simulink model "model"  (R2024b)
settings: Solver=FixedStepAuto  StartTime=0  StopTime=12000  FixedStep=1  RelTol=1e-3
model workspace (MAT data in the model file):
  initial_altitude = 418
  initial_latitude = 48
  initial_longitude = 11
  updraft_locations = [48.9421342125 12.8571640345]
values from neighbouring files (symbols this model uses):
  sounding_buses = [sounding_buses, new_bus]    [create_bus.m]
  updrafts = cell(1, num_updrafts)    [test_thermal_model.m]
libraries: matrix_library x2, aerolibtransform2 x2, aerolibanim x1
settings Model: Creator=ge59guz  LastModifiedBy=Pedro
settings DebuggingCC: UnconnectedInputMsg=warning  UnconnectedOutputMsg=warning  UnconnectedLineMsg=warning
settings ModelReferenceCC: EnableRefExpFcnMdlSchedulingChecks=on
settings SFSimCC: LegacyBehaviorForPersistentVarInContinuousTime=on
settings RTWCC: GPUComputeCapability=3.5  DLArmComputeVersion=19.05

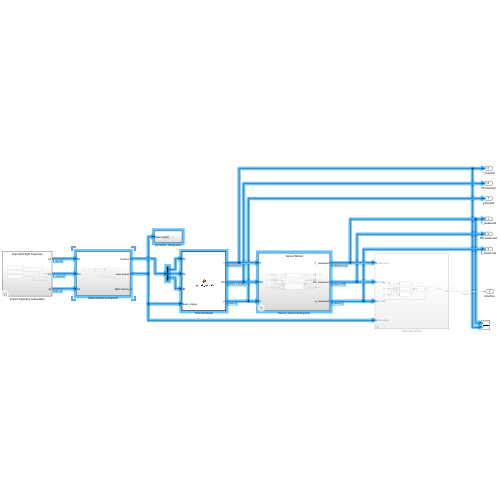
[thumbnail: Simulink's stored preview of the top-level diagram]
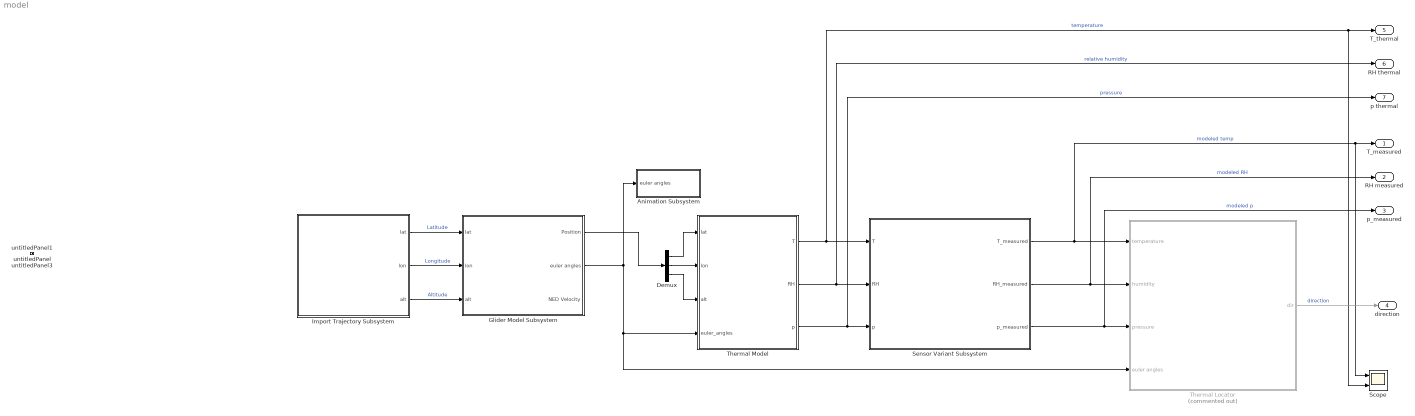
== system model ==
  Animation Subsystem : Subsystem
  Demux : Demux  Outputs=3
  Glider Model Subsystem : Subsystem
  Import Trajectory Subsystem : Subsystem  Variant=on
  Scope : Scope  NumInputPorts=2
  Sensor Variant Subsystem : Subsystem  Variant=on
  Thermal Locator : Subsystem  Commented=on
  Thermal Model : MATLAB Function  TreatAsAtomicUnit=on
  untitledPanel : Subsystem  Tag=HiddenForWebPanel  IsWebBlockPanel=on
  untitledPanel1 : Subsystem  Tag=HiddenForWebPanel  IsWebBlockPanel=on
  untitledPanel3 : Subsystem  Tag=HiddenForWebPanel  IsWebBlockPanel=on
  T_measured : Outport
  RH measured : Outport  Port=2
  p_measured : Outport  Port=3
  direction : Outport  Port=4
  T_thermal : Outport  Port=5
  RH thermal : Outport  Port=6
  p thermal : Outport  Port=7
  wires:
  Thermal Model/1(T) -> Sensor Variant Subsystem/1(T), Scope/2, T_thermal/1  "temperature"
  Thermal Model/3(p) -> p thermal/1, Sensor Variant Subsystem/3(p)  "pressure"
  Import Trajectory Subsystem/1(lat) -> Glider Model Subsystem/1(lat)  "Latitude"
  Import Trajectory Subsystem/2(lon) -> Glider Model Subsystem/2(lon)  "Longitude"
  Sensor Variant Subsystem/1(T_measured) -> Thermal Locator/1(temperature), Scope/1, T_measured/1  "modeled temp"
  Sensor Variant Subsystem/2(RH_measured) -> Thermal Locator/2(humidity), RH measured/1  "modeled RH"
  Sensor Variant Subsystem/3(p_measured) -> Thermal Locator/3(pressure), p_measured/1  "modeled p"
  Thermal Model/2(RH) -> Sensor Variant Subsystem/2(RH), RH thermal/1  "relative humidity"
  Import Trajectory Subsystem/3(alt) -> Glider Model Subsystem/3(alt)  "Altitude"
  Glider Model Subsystem/2(euler angles) -> Animation Subsystem/1(euler angles), Thermal Locator/4(euler angles), Thermal Model/4(euler_angles)
  Glider Model Subsystem/1(Position) -> Demux/1
  Demux/1 -> Thermal Model/1(lat)
  Demux/2 -> Thermal Model/2(lon)
  Demux/3 -> Thermal Model/3(alt)
  Thermal Locator/1(dir) -> direction/1  "direction"

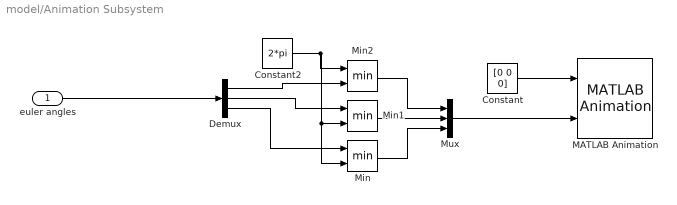
== system model/Animation Subsystem ==
  euler angles : Inport
  Constant : Constant  Value=[0 0 0]
  Constant2 : Constant  Value=2*pi
  Demux : Demux  Outputs=3
  MATLAB Animation : aerolibanim/MATLAB Animation  Tag=Matlab Animation 6 DOF  Vehicles=1  Geometries='pa24-250_orange.ac'  BoundingBoxCoordinates=[-50,50,-50,50,-50,50]  CameraOffset=[-150,-50,0]  CameraViewAngle=3  SampleTime=2  FigurePosition=[6.416667e+02,3.616667e+02,6.386667e+02,3.033333e+02]
  Min : MinMax  Inputs=2
  Min1 : MinMax  Inputs=2
  Min2 : MinMax  Inputs=2
  Mux : Mux  Inputs=3
  wires:
  Demux/3 -> Min/1
  Demux/2 -> Min1/1
  Demux/1 -> Min2/2
  Min2/1 -> Mux/1
  Min/1 -> Mux/3
  Min1/1 -> Mux/2
  euler angles/1 -> Demux/1
  Constant2/1 -> Min/2, Min1/2, Min2/1
  Constant/1 -> MATLAB Animation/1
  Mux/1 -> MATLAB Animation/2

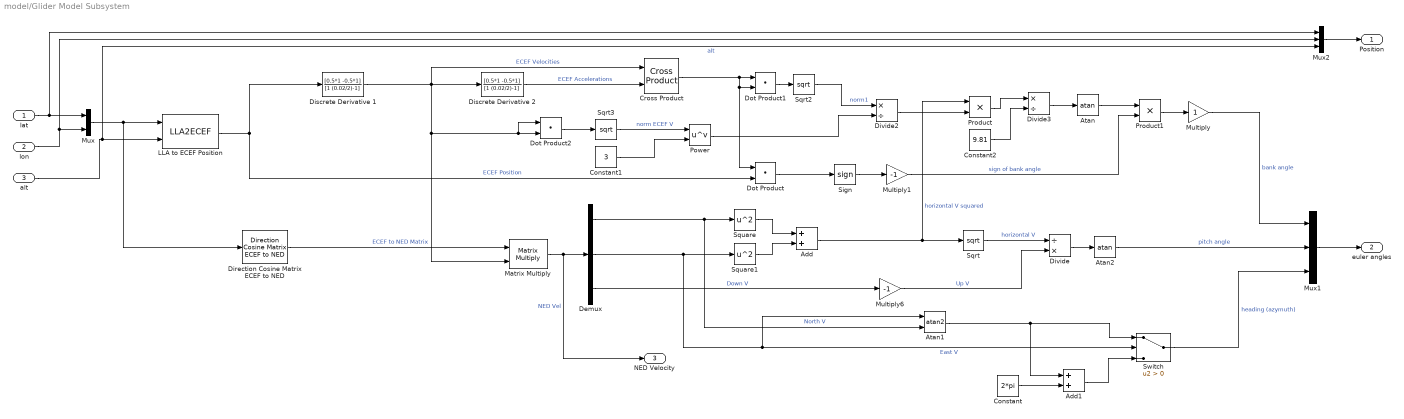
== system model/Glider Model Subsystem ==
  lat : Inport
  lon : Inport  Port=2
  alt : Inport  Port=3
  Add : Sum
  Add1 : Sum
  Atan : Trigonometry  Operator=atan
  Atan1 : Trigonometry  Operator=atan2
  Atan2 : Trigonometry  Operator=atan
  Constant : Constant  Value=2*pi
  Constant1 : Constant  Value=3
  Constant2 : Constant  Value=9.81
  Cross Product : matrix_library/Cross Product
  Demux : Demux  Outputs=3
  Direction Cosine Matrix ECEF to NED : aerolibtransform2/Direction Cosine Matrix ECEF to NED
  Discrete Derivative 1 : DiscreteTransferFcn  Numerator=[0.5*1 -0.5*1]  Denominator=[1 (0.02/2)-1]
  Discrete Derivative 2 : DiscreteTransferFcn  Numerator=[0.5*1 -0.5*1]  Denominator=[1 (0.02/2)-1]
  Divide : Product  Inputs=/*
  Divide2 : Product  Inputs=*/
  Divide3 : Product  Inputs=*/
  Dot Product : DotProduct  OutDataTypeStr=Inherit: Inherit via internal rule
  Dot Product1 : DotProduct  OutDataTypeStr=Inherit: Inherit via internal rule
  Dot Product2 : DotProduct  OutDataTypeStr=Inherit: Inherit via internal rule
  LLA to ECEF Position : LLA2ECEF
  Matrix Multiply : Product  Multiplication=Matrix(*)
  Multiply : Gain
  Multiply1 : Gain  Gain=-1
  Multiply6 : Gain  Gain=-1
  Mux : Mux  Inputs=2
  Mux1 : Mux  Inputs=3
  Mux2 : Mux  Inputs=3
  Power : Math  Operator=pow
  Product : Product
  Product1 : Product
  Sign : Signum
  Sqrt : Sqrt
  Sqrt2 : Sqrt
  Sqrt3 : Sqrt
  Square : Math  Operator=square
  Square1 : Math  Operator=square
  Switch : Switch  Criteria=u2 > Threshold  SaturateOnIntegerOverflow=off  InputSameDT=off
  Position : Outport
  euler angles : Outport  Port=2
  NED Velocity : Outport  Port=3
  wires:
  lon/1 -> Mux2/2, Mux/2
  lat/1 -> Mux2/1, Mux/1
  Mux/1 -> Direction Cosine Matrix ECEF to NED/1, LLA to ECEF Position/1
  alt/1 -> Mux2/3, LLA to ECEF Position/2  "alt"
  Direction Cosine Matrix ECEF to NED/1 -> Matrix Multiply/1  "ECEF to NED Matrix"
  LLA to ECEF Position/1 -> Dot Product/2, Discrete Derivative 1/1  "ECEF Position"
  Discrete Derivative 1/1 -> Matrix Multiply/2, Dot Product2/1, Dot Product2/2, Discrete Derivative 2/1, Cross Product/1  "ECEF Velocities"
  Matrix Multiply/1 -> NED Velocity/1, Demux/1  "NED Vel"
  Demux/2 -> Square1/1, Atan1/1, Switch/2  "East V"
  Demux/1 -> Atan1/2, Square/1  "North V"
  Square/1 -> Add/1
  Add/1 -> Sqrt/1, Product/1  "horizontal V squared"
  Cross Product/1 -> Dot Product/1, Dot Product1/2, Dot Product1/1
  Dot Product2/1 -> Sqrt3/1
  Sqrt3/1 -> Power/1  "norm ECEF V"
  Constant1/1 -> Power/2
  Sqrt2/1 -> Divide2/1  "norm1"
  Power/1 -> Divide2/2
  Divide2/1 -> Product/2
  Product/1 -> Divide3/1
  Constant2/1 -> Divide3/2
  Divide3/1 -> Atan/1
  Atan/1 -> Product1/1
  Multiply/1 -> Mux1/1  "bank angle"
  Dot Product/1 -> Sign/1
  Sign/1 -> Multiply1/1
  Product1/1 -> Multiply/1
  Dot Product1/1 -> Sqrt2/1
  Multiply1/1 -> Product1/2  "sign of bank angle"
  Square1/1 -> Add/2
  Constant/1 -> Add1/2
  Atan1/1 -> Add1/1, Switch/1
  Add1/1 -> Switch/3
  Switch/1 -> Mux1/3  "heading (azymuth)"
  Sqrt/1 -> Divide/1  "horizontal V"
  Divide/1 -> Atan2/1
  Demux/3 -> Multiply6/1  "Down V"
  Atan2/1 -> Mux1/2  "pitch angle"
  Multiply6/1 -> Divide/2  "Up V"
  Mux1/1 -> euler angles/1
  Discrete Derivative 2/1 -> Cross Product/2  "ECEF Accelerations"
  Mux2/1 -> Position/1

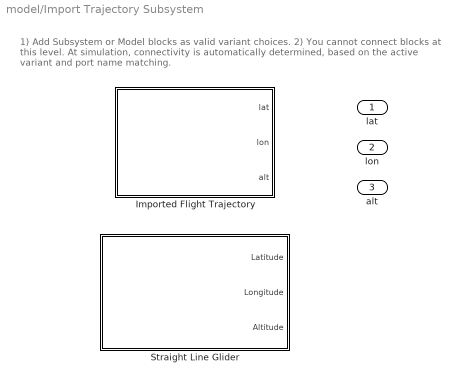
== system model/Import Trajectory Subsystem ==
  note: 1) Add Subsystem or Model blocks as valid variant choices.
      | 2) You cannot connect blocks at this level. At simulation, connectivity is automatically
      | determined, based on the active variant and port name matching.
  Imported Flight Trajectory : Subsystem  VariantControl=true
  Straight Line Glider : Subsystem  VariantControl=false
  lat : Outport
  lon : Outport  Port=2
  alt : Outport  Port=3

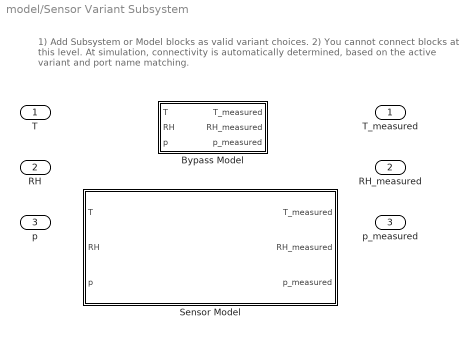
== system model/Sensor Variant Subsystem ==
  note: 1) Add Subsystem or Model blocks as valid variant choices.
      | 2) You cannot connect blocks at this level. At simulation, connectivity is automatically
      | determined, based on the active variant and port name matching.
  T : Inport
  RH : Inport  Port=2
  p : Inport  Port=3
  Bypass Model : Subsystem  VariantControl=false
  Sensor Model : Subsystem  VariantControl=true
  T_measured : Outport
  RH_measured : Outport  Port=2
  p_measured : Outport  Port=3

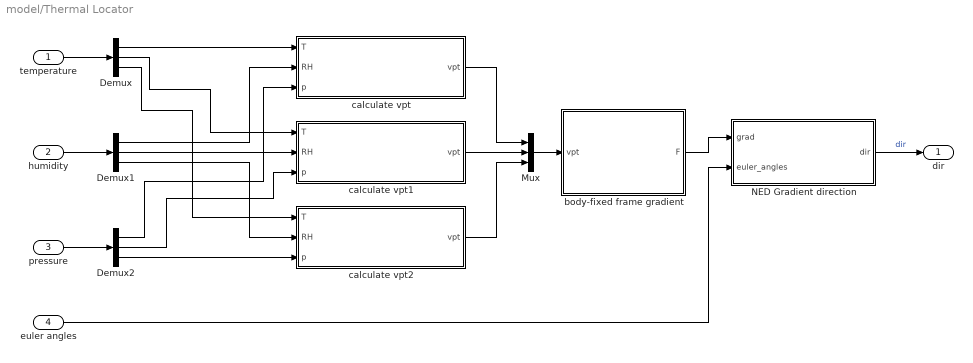
== system model/Thermal Locator ==
  temperature : Inport
  humidity : Inport  Port=2
  pressure : Inport  Port=3
  euler angles : Inport  Port=4
  Demux : Demux  Outputs=3
  Demux1 : Demux  Outputs=3
  Demux2 : Demux  Outputs=3
  Mux : Mux  Inputs=3
  NED Gradient direction : MATLAB Function  TreatAsAtomicUnit=on
  body-fixed frame gradient : MATLAB Function  TreatAsAtomicUnit=on
  calculate vpt : MATLAB Function  TreatAsAtomicUnit=on
  calculate vpt1 : MATLAB Function  TreatAsAtomicUnit=on
  calculate vpt2 : MATLAB Function  TreatAsAtomicUnit=on
  dir : Outport
  wires:
  temperature/1 -> Demux/1
  Demux/1 -> calculate vpt/1(T)
  Demux/2 -> calculate vpt1/1(T)
  Demux/3 -> calculate vpt2/1(T)
  humidity/1 -> Demux1/1
  Demux1/1 -> calculate vpt/2(RH)
  Demux1/2 -> calculate vpt1/2(RH)
  Demux1/3 -> calculate vpt2/2(RH)
  pressure/1 -> Demux2/1
  Demux2/1 -> calculate vpt/3(p)
  Demux2/2 -> calculate vpt1/3(p)
  Demux2/3 -> calculate vpt2/3(p)
  calculate vpt/1(vpt) -> Mux/1
  calculate vpt1/1(vpt) -> Mux/2
  calculate vpt2/1(vpt) -> Mux/3
  Mux/1 -> body-fixed frame gradient/1(vpt)
  body-fixed frame gradient/1(F) -> NED Gradient direction/1(grad)
  euler angles/1 -> NED Gradient direction/2(euler_angles)
  NED Gradient direction/1(dir) -> dir/1  "dir"

== system model/untitledPanel ==
  panelInfo : PanelWebBlock  Tag=HiddenForWebPanel  PanelInfo="{\"compacted\":true,\"height\":246,\"isActiveTab\":false,\"labels\":{\"label1365784696\":{\"deleted\":false,\"left\":18,\"settings\":{\"backgroundColor\":\"rgba(0, 0, 0, 0)\",\"bold\":false,\"font\":\"Arial\",\"fontColor\":\"black\",\"fontSize\":0.91,\"italicized\":false,\"underlined\":false},\"text\":\"Lifting condensation level:\",\"top\":138},\"label2522607047\":{\"deleted\":false,\"left\":20,\"settings\":{\"backgroundColor\":\"rgba(0, 0, 0, 0)\",\"bold\":false,\"font\":\"Arial\",\"fontColor\":\"black\",\"fontSize\":0.91,\"italicized\":false,\"underlined\":false},\"text\":\"Sounding location:\",\"top\":61},\"label6819632646\":{\"deleted\":false,\"left\":18,\"settings\":{\"backgroundColor\":\"rgba(0, 0, 0, 0)\",\"bold\":false,\"font\":\"Arial\",\"fontColor\":\"black\",\"fontSize\":0.91,\"italicized\":false,\"underlined\":false},\"text\":\"Mixed layer height:\",\"top\":100},\"label7929561413\":{\"deleted\":false,\"left\":18,\"settings\":{\"backgroundColor\":\"rgba(0, 0, 0, 0)\",\"bold\":false,\"font\":\"Arial\",\"fontColor\":\"black\",\"fontSize\":0.91,\"italicized\":false,\"underlined\":false},\"text\":\"Sounding date:\",\"top\":22}},\"left\":1938,\"name\":\"Sounding\",\"panelId\":\"panelId-b7bbacb4-b1f5-40a6-a59f-f1281bc15f19\",\"tabIndex\":2,\"tabbedSetId\":\"tabbedSet2696921389\",\"top\":7,\"type\":\"panel\",\"version\":\"2019b\",\"visible\":false,\"width\":464,\"zIndex\":1500006}"  PanelSnapshot=<binary blob, 23204 chars, not shown>

== system model/untitledPanel1 ==
  Climb : EditField  Tag=HiddenForWebPanel  PanelInfo="{\"height\":33,\"left\":126,\"panelId\":\"panelId-a8974220-6362-43f7-be10-4c2880e9e60b\",\"top\":107,\"type\":\"panelChild\",\"version\":\"2019b\",\"width\":46,\"zIndex\":1500006}"  LabelPosition=Hide  ShowInitialText=on  Alignment=Center
  Heading : EditField  Tag=HiddenForWebPanel  PanelInfo="{\"height\":31,\"left\":125,\"panelId\":\"panelId-a8974220-6362-43f7-be10-4c2880e9e60b\",\"top\":69,\"type\":\"panelChild\",\"version\":\"2019b\",\"width\":46,\"zIndex\":1500004}"  LabelPosition=Hide  ShowInitialText=on  Alignment=Center
  panelInfo : PanelWebBlock  Tag=HiddenForWebPanel  PanelInfo="{\"compacted\":true,\"height\":223,\"isActiveTab\":true,\"labels\":{\"label0009524542\":{\"deleted\":false,\"left\":132,\"settings\":{\"backgroundColor\":\"rgba(0, 0, 0, 0)\",\"bold\":false,\"font\":\"Arial\",\"fontColor\":\"black\",\"fontSize\":0.82,\"italicized\":false,\"underlined\":false},\"text\":\"alt\",\"top\":167},\"label0163547761\":{\"deleted\":false,\"left\":23,\"settings\":{\"backgroundColor\":\"rgba(0, 0, 0, 0)\",\"bold\":false,\"font\":\"Arial\",\"fontColor\":\"black\",\"fontSize\":0.82,\"italicized\":false,\"underlined\":false},\"text\":\"lat\",\"top\":167},\"label2478146783\":{\"deleted\":false,\"left\":11,\"settings\":{\"backgroundColor\":\"rgba(0, 0, 0, 0)\",\"bold\":false,\"font\":\"Arial\",\"fontColor\":\"black\",\"fontSize\":0.82,\"italicized\":false,\"underlined\":false},\"text\":\"climb angle (deg)\",\"top\":116},\"label4468598914\":{\"deleted\":false,\"left\":10,\"settings\":{\"backgroundColor\":\"rgba(0, 0, 0, 0)\",\"bold\":false,\"font\":\"Arial\",\"fontColor\":\"black\",\"fontSize\":0.82,\"italicized\":false,\"underlined\":false},\"text\":\"heading (deg)\",\"top\":77},\"label4953567006\":{\"deleted\":false,\"left\":9,\"settings\":{\"backgroundColor\":\"rgba(0, 0, 0, 0)\",\"bold\":false,\"font\":\"Arial\",\"fontColor\":\"black\",\"fontSize\":0.82,\"italicized\":false,\"underlined\":false},\"text\":\"initial velocity (m\\/s)\",\"top\":39},\"label6880872590\":{\"deleted\":false,\"left\":74,\"settings\":{\"backgroundColor\":\"rgba(0, 0, 0, 0)\",\"bold\":false,\"font\":\"Arial\",\"fontColor\":\"black\",\"fontSize\":0.82,\"italicized\":false,\"underlined\":false},\"text\":\"lon\",\"top\":167},\"label9788082855\":{\"deleted\":false,\"left\":12,\"settings\":{\"backgroundColor\":\"rgba(0, 0, 0, 0)\",\"bold\":true,\"font\":\"Arial\",\"fontColor\":\"black\",\"fontSize\":0.82,\"italicized\":false,\"underlined\":false},\"text\":\"Inputs\",\"top\":9},\"label9797548924\":{\"deleted\":false,\"left\":13,\"settings\":{\"backgroundColor\":\"rgba(0, 0, 0, 0)\",\"bold\":false,\"font\":\"Arial\",\"fontColor\":\"black\",\"fontSize\":0.82,\"italicized\":false,\"underlined\":false},\"text\":\"initial position (deg, m)\",\"top\":147}},\"left\":1938,\"name\":\"Glider\",\"panelId\":\"panelId-a8974220-6362-43f7-be10-4c2880e9e60b\",\"tabIndex\":0,\"tabbedSetId\":\"tabbedSet2696921389\",\"top\":7,\"type\":\"panel\",\"version\":\"2019b\",\"visible\":true,\"width\":484,\"zIndex\":1500004}"  PanelSnapshot=<binary blob, 27484 chars, not shown>
  velocity : EditField  Tag=HiddenForWebPanel  PanelInfo="{\"height\":33,\"left\":124,\"panelId\":\"panelId-a8974220-6362-43f7-be10-4c2880e9e60b\",\"top\":31,\"type\":\"panelChild\",\"version\":\"2019b\",\"width\":47,\"zIndex\":1500002}"  LabelPosition=Hide  ShowInitialText=on  Alignment=Center

== system model/untitledPanel3 ==
  Callback Button : CustomCallbackButton  Tag=HiddenForWebPanel  PanelInfo="{\"height\":50,\"left\":66,\"panelId\":\"panelId-5dd198ca-f2e6-4c37-9029-21f4a79994a1\",\"top\":24,\"type\":\"panelChild\",\"version\":\"2019b\",\"width\":142,\"zIndex\":1500002}"  Configuration="{\"components\":[{\"name\":\"BackgroundImageComponent\",\"settings\":{\"image\":{\"size\":[0,0],\"src\":\"default\",\"srcOrientation\":\"Right\"},\"position\":[0,0,1,1]}},{\"name\":\"ButtonStateComponent\",\"settings\":{\"buttonType\":\"momentary\",\"clickFcn\":\"[filename,filepath] = uigetfile({'*.igc';'*.mat'});\\n\\nif filename == 0\\n    return\\nelseif contains(filename, '.igc')\\n    % Parse igc file\\n    [flight, name] = parse_igc_file([filepath filename]);\\n    % Save flight to a .mat file\\n    save(strcat('Flights\\/',name, '.mat'), 'flight');\\nelseif contains(filename, '.mat')\\n    % Open saved flight\\n    load([filepath filename]);\\nelse\\n    return\\nend\\n\",\"latched\":false,\"offValue\":null,\"onValue\":1,\"position\":[0,0,1,1],\"pressDelay\":\"500\",\"pressFcn\":\"\",\"repeatInterval\":\"0\",\"states\":[{\"horizontalAlignment\":\"center\",\"image\":{\"position\":[0,0,1,1],\"size\":[1,1],\"src\":\"default\",\"srcOrientation\":\"Right\"},\"label\":{\"color\":[0.01176470588,0.01176470588,0.01176470588,1],\"icon\":{\"size\":[0,0],\"src\":\"default\",\"srcOrientation\":\"Right\"},\"iconPlacement\":\"left\",\"opacity\":1,\"show\":true,\"text\":{\"content\":\"Load flight\",\"font\":\"Helvetica\"}},\"labelOffset\":[0,0],\"verticalAlignment\":\"middle\"},{\"horizontalAlignment\":\"center\",\"image\":{\"position\":[0,0,1,1],\"size\":[1,1],\"src\":\"default\",\"srcOrientation\":\"Right\"},\"label\":{\"color\":[0.01176470588,0.01176470588,0.01176470588,1],\"icon\":{\"size\":[0,0],\"src\":\"default\",\"srcOrientation\":\"Right\"},\"iconPlacement\":\"left\",\"opacity\":1,\"show\":true,\"text\":{\"content\":\"Load flight\",\"font\":\"Helvetica\"}},\"labelOffset\":[0,0],\"verticalAlignment\":\"middle\"},{\"horizontalAlignment\":\"center\",\"image\":{\"position\":[0,0,1,1],\"size\":[1,1],\"src\":\"default\",\"srcOrientation\":\"Right\"},\"label\":{\"color\":[0.01176470588,0.01176470588,0.01176470588,1],\"icon\":{\"size\":[0,0],\"src\":\"default\",\"srcOrientation\":\"Right\"},\"iconPlacement\":\"left\",\"opacity\":1,\"show\":true,\"text\":{\"content\":\"Load flight\",\"font\":\"Helvetica\"}},\"labelOffset\":[0,0],\"verticalAlignment\":\"middle\"},{\"horizontalAlignment\":\"center\",\"image\":{\"position\":[0,0,1,1],\"size\":[1,1],\"src\":\"default\",\"srcOrientation\":\"Right\"},\"label\":{\"color\":[0.01176470588,0.01176470588,0.01176470588,1],\"icon\":{\"size\":[0,0],\"src\":\"default\",\"srcOrientation\":\"Right\"},\"iconPlacement\":\"left\",\"opacity\":1,\"show\":true,\"text\":{\"content\":\"Load flight\",\"font\":\"Helvetica\"}},\"labelOffset\":[0,0],\"verticalAlignment\":\"middle\"}]}},{\"name\":\"ForegroundImageComponent\",\"settings\":{\"image\":{\"size\":[0,0],\"src\":\"default\",\"srcOrientation\":\"Right\"},\"isForeground\":1,\"position\":[0,0,1,1]}}],\"settings\":{\"BindingType\":\"standalone\",\"backgroundColor\":[244,244,244,1],\"backgroundOffset\":0.2,\"backgroundOpacity\":1,\"fixedAspectRatio\":\"off\",\"foregroundColor\":[0.01176470588,0.01176470588,0.01176470588,1],\"migratedFromLegacy\":true,\"useBackgroundColor\":true,\"variant\":\"callback\",\"version\":\"R2024b\"},\"type\":\"Button\"}"  CustomBackgroundColor="{\"color\":[0.9568627451,0.9568627451,0.9568627451],\"show\":true}"
  Callback Button1 : CustomCallbackButton  Tag=HiddenForWebPanel  PanelInfo="{\"height\":47,\"left\":62,\"panelId\":\"panelId-5dd198ca-f2e6-4c37-9029-21f4a79994a1\",\"top\":89,\"type\":\"panelChild\",\"version\":\"2019b\",\"width\":149,\"zIndex\":1499998}"  Configuration="{\"components\":[{\"name\":\"BackgroundImageComponent\",\"settings\":{\"image\":{\"size\":[0,0],\"src\":\"default\",\"srcOrientation\":\"Right\"},\"position\":[0,0,1,1]}},{\"name\":\"ButtonStateComponent\",\"settings\":{\"buttonType\":\"momentary\",\"clickFcn\":\"display_chart(flight.trajectory,stations);\",\"onValue\":1,\"position\":[0,0,1,1],\"pressDelay\":\"500\",\"pressFcn\":\"\",\"repeatInterval\":\"0\",\"states\":[{\"horizontalAlignment\":\"center\",\"image\":{\"position\":[0,0,1,1],\"size\":[1,1],\"src\":\"default\",\"srcOrientation\":\"Right\"},\"label\":{\"color\":[0.01176470588,0.01176470588,0.01176470588,1],\"icon\":{\"size\":[0,0],\"src\":\"default\",\"srcOrientation\":\"Right\"},\"iconPlacement\":\"left\",\"opacity\":1,\"show\":true,\"text\":{\"content\":\"Place updrafts\",\"font\":\"Helvetica\"}},\"labelOffset\":[0,0],\"verticalAlignment\":\"middle\"},{\"horizontalAlignment\":\"center\",\"image\":{\"position\":[0,0,1,1],\"size\":[1,1],\"src\":\"default\",\"srcOrientation\":\"Right\"},\"label\":{\"color\":[0.01176470588,0.01176470588,0.01176470588,1],\"icon\":{\"size\":[0,0],\"src\":\"default\",\"srcOrientation\":\"Right\"},\"iconPlacement\":\"left\",\"opacity\":1,\"show\":true,\"text\":{\"content\":\"Place updrafts\",\"font\":\"Helvetica\"}},\"labelOffset\":[0,0],\"verticalAlignment\":\"middle\"},{\"horizontalAlignment\":\"center\",\"image\":{\"position\":[0,0,1,1],\"size\":[1,1],\"src\":\"default\",\"srcOrientation\":\"Right\"},\"label\":{\"color\":[0.01176470588,0.01176470588,0.01176470588,1],\"icon\":{\"size\":[0,0],\"src\":\"default\",\"srcOrientation\":\"Right\"},\"iconPlacement\":\"left\",\"opacity\":1,\"show\":true,\"text\":{\"content\":\"Place updrafts\",\"font\":\"Helvetica\"}},\"labelOffset\":[0,0],\"verticalAlignment\":\"middle\"},{\"horizontalAlignment\":\"center\",\"image\":{\"position\":[0,0,1,1],\"size\":[1,1],\"src\":\"default\",\"srcOrientation\":\"Right\"},\"label\":{\"color\":[0.01176470588,0.01176470588,0.01176470588,1],\"icon\":{\"size\":[0,0],\"src\":\"default\",\"srcOrientation\":\"Right\"},\"iconPlacement\":\"left\",\"opacity\":1,\"show\":true,\"text\":{\"content\":\"Place updrafts\",\"font\":\"Helvetica\"}},\"labelOffset\":[0,0],\"verticalAlignment\":\"middle\"}]}},{\"name\":\"ForegroundImageComponent\",\"settings\":{\"image\":{\"size\":[0,0],\"src\":\"default\",\"srcOrientation\":\"Right\"},\"isForeground\":1,\"position\":[0,0,1,1]}}],\"settings\":{\"BindingType\":\"standalone\",\"backgroundColor\":[244,244,244,1],\"backgroundOffset\":0.2,\"backgroundOpacity\":1,\"fixedAspectRatio\":\"off\",\"foregroundColor\":[0.01176470588,0.01176470588,0.01176470588,1],\"migratedFromLegacy\":true,\"useBackgroundColor\":true,\"variant\":\"callback\",\"version\":\"R2024b\"},\"type\":\"Button\"}"  CustomBackgroundColor="{\"color\":[0.9568627451,0.9568627451,0.9568627451],\"show\":true}"
  panelInfo : PanelWebBlock  Tag=HiddenForWebPanel  PanelInfo="{\"compacted\":true,\"height\":231,\"isActiveTab\":false,\"left\":1938,\"name\":\"Flight\",\"panelId\":\"panelId-5dd198ca-f2e6-4c37-9029-21f4a79994a1\",\"tabIndex\":1,\"tabbedSetId\":\"tabbedSet2696921389\",\"top\":7,\"type\":\"panel\",\"version\":\"2019b\",\"visible\":false,\"width\":437,\"zIndex\":1500010}"  PanelSnapshot=<binary blob, 11188 chars, not shown>

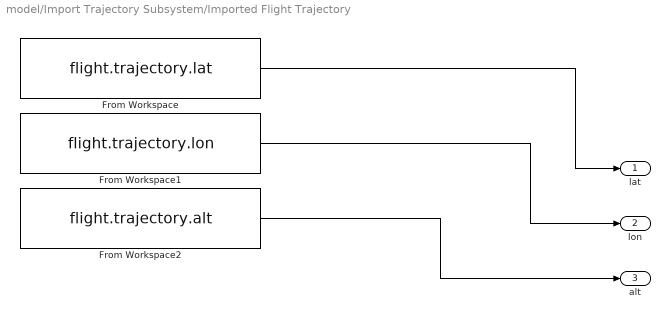
== system model/Import Trajectory Subsystem/Imported Flight Trajectory ==
  From Workspace : FromWorkspace  VariableName=flight.trajectory.lat  ZeroCross=off  OutputAfterFinalValue=Holding final value
  From Workspace1 : FromWorkspace  VariableName=flight.trajectory.lon  ZeroCross=off  OutputAfterFinalValue=Holding final value
  From Workspace2 : FromWorkspace  VariableName=flight.trajectory.alt  ZeroCross=off  OutputAfterFinalValue=Holding final value
  lat : Outport
  lon : Outport  Port=2
  alt : Outport  Port=3
  wires:
  From Workspace1/1 -> lon/1
  From Workspace/1 -> lat/1
  From Workspace2/1 -> alt/1

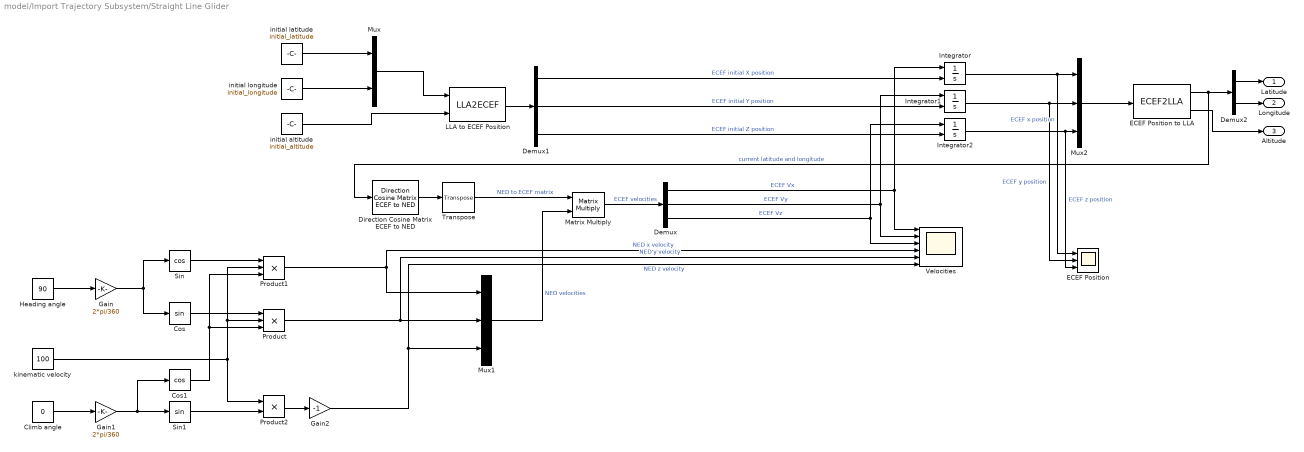
== system model/Import Trajectory Subsystem/Straight Line Glider ==
  Climb angle : Constant  Value=0
  Cos : Trigonometry  OutputSignalType=real
  Cos1 : Trigonometry  Operator=cos
  Demux : Demux  Outputs=3
  Demux1 : Demux  Outputs=3
  Demux2 : Demux  Outputs=2
  Direction Cosine Matrix ECEF to NED : aerolibtransform2/Direction Cosine Matrix ECEF to NED
  ECEF Position : Scope  NumInputPorts=3
  ECEF Position to LLA : ECEF2LLA
  Gain : Gain  Gain=2*pi/360
  Gain1 : Gain  Gain=2*pi/360
  Gain2 : Gain  Gain=-1
  Heading angle : Constant  Value=90
  Integrator : Integrator  InitialConditionSource=external
  Integrator1 : Integrator  InitialConditionSource=external
  Integrator2 : Integrator  InitialConditionSource=external
  LLA to ECEF Position : LLA2ECEF
  Matrix Multiply : Product  Multiplication=Matrix(*)
  Mux : Mux  Inputs=2
  Mux1 : Mux  Inputs=3
  Mux2 : Mux  Inputs=3
  Product : Product  Inputs=3
  Product1 : Product  Inputs=3
  Product2 : Product
  Sin : Trigonometry  Operator=cos  OutputSignalType=real
  Sin1 : Trigonometry  OutputSignalType=real
  Transpose : matrix_library/Transpose
  Velocities : Scope  NumInputPorts=6
  initial altitude : Constant  Value=initial_altitude
  initial latitude : Constant  Value=initial_latitude
  initial longitude : Constant  Value=initial_longitude
  kinematic velocity : Constant  Value=100
  Latitude : Outport  Unit=deg  PortDimensions=1
  Longitude : Outport  Port=2  Unit=deg  PortDimensions=1
  Altitude : Outport  Port=3  Unit=m  PortDimensions=1
  wires:
  Integrator1/1 -> Mux2/2, ECEF Position/2  "ECEF y position"
  Integrator/1 -> Mux2/1, ECEF Position/1  "ECEF x position"
  Integrator2/1 -> ECEF Position/3, Mux2/3  "ECEF z position"
  Product2/1 -> Gain2/1
  Mux1/1 -> Matrix Multiply/2  "NED velocities"
  Matrix Multiply/1 -> Demux/1  "ECEF velocities"
  kinematic velocity/1 -> Product2/1, Product1/2, Product/2
  Sin1/1 -> Product2/2
  Cos/1 -> Product/1
  Gain2/1 -> Velocities/6, Mux1/3  "NED z velocity"
  Gain/1 -> Sin/1, Cos/1
  Heading angle/1 -> Gain/1
  Gain1/1 -> Cos1/1, Sin1/1
  Product/1 -> Velocities/5, Mux1/2  "NED y velocity"
  Direction Cosine Matrix ECEF to NED/1 -> Transpose/1
  Climb angle/1 -> Gain1/1
  Cos1/1 -> Product1/3, Product/3
  initial longitude/1 -> Mux/2
  initial latitude/1 -> Mux/1
  Mux/1 -> LLA to ECEF Position/1
  Product1/1 -> Mux1/1, Velocities/4  "NED x velocity"
  Sin/1 -> Product1/1
  Transpose/1 -> Matrix Multiply/1  "NED to ECEF matrix"
  initial altitude/1 -> LLA to ECEF Position/2
  Demux/1 -> Velocities/1, Integrator/1  "ECEF Vx"
  Demux/2 -> Velocities/2, Integrator1/1  "ECEF Vy"
  Demux/3 -> Integrator2/1, Velocities/3  "ECEF Vz"
  LLA to ECEF Position/1 -> Demux1/1
  Demux1/1 -> Integrator/2  "ECEF initial X position"
  Demux1/2 -> Integrator1/2  "ECEF initial Y position"
  Demux1/3 -> Integrator2/2  "ECEF initial Z position"
  Mux2/1 -> ECEF Position to LLA/1
  ECEF Position to LLA/1 -> Demux2/1, Direction Cosine Matrix ECEF to NED/1  "current latitude and longitude"
  Demux2/1 -> Latitude/1
  Demux2/2 -> Longitude/1
  ECEF Position to LLA/2 -> Altitude/1

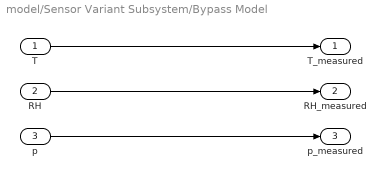
== system model/Sensor Variant Subsystem/Bypass Model ==
  T : Inport
  RH : Inport  Port=2
  p : Inport  Port=3
  T_measured : Outport
  RH_measured : Outport  Port=2
  p_measured : Outport  Port=3
  wires:
  T/1 -> T_measured/1
  RH/1 -> RH_measured/1
  p/1 -> p_measured/1

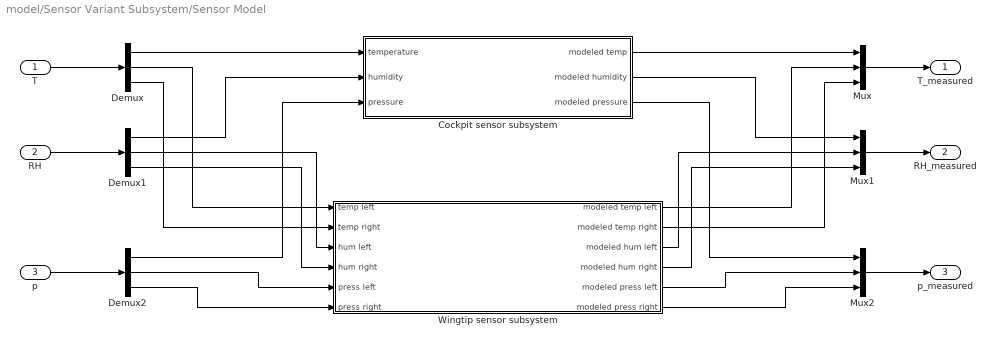
== system model/Sensor Variant Subsystem/Sensor Model ==
  T : Inport
  RH : Inport  Port=2
  p : Inport  Port=3
  Cockpit sensor subsystem : Subsystem
  Demux : Demux  Outputs=3
  Demux1 : Demux  Outputs=3
  Demux2 : Demux  Outputs=3
  Mux : Mux  Inputs=3
  Mux1 : Mux  Inputs=3
  Mux2 : Mux  Inputs=3
  Wingtip sensor subsystem : Subsystem
  T_measured : Outport
  RH_measured : Outport  Port=2
  p_measured : Outport  Port=3
  wires:
  RH/1 -> Demux1/1
  T/1 -> Demux/1
  Mux/1 -> T_measured/1
  Mux1/1 -> RH_measured/1
  Demux1/1 -> Cockpit sensor subsystem/2(humidity)
  Demux1/2 -> Wingtip sensor subsystem/3(hum left)
  Demux1/3 -> Wingtip sensor subsystem/4(hum right)
  Demux/1 -> Cockpit sensor subsystem/1(temperature)
  Cockpit sensor subsystem/1(modeled temp) -> Mux/1
  Demux/2 -> Wingtip sensor subsystem/1(temp left)
  Demux/3 -> Wingtip sensor subsystem/2(temp right)
  Wingtip sensor subsystem/1(modeled temp left) -> Mux/2
  Wingtip sensor subsystem/2(modeled temp right) -> Mux/3
  p/1 -> Demux2/1
  Demux2/1 -> Cockpit sensor subsystem/3(pressure)
  Cockpit sensor subsystem/2(modeled humidity) -> Mux1/1
  Demux2/2 -> Wingtip sensor subsystem/5(press left)
  Demux2/3 -> Wingtip sensor subsystem/6(press right)
  Wingtip sensor subsystem/3(modeled hum left) -> Mux1/2
  Wingtip sensor subsystem/4(modeled hum right) -> Mux1/3
  Wingtip sensor subsystem/5(modeled press left) -> Mux2/2
  Wingtip sensor subsystem/6(modeled press right) -> Mux2/3
  Cockpit sensor subsystem/3(modeled pressure) -> Mux2/1
  Mux2/1 -> p_measured/1

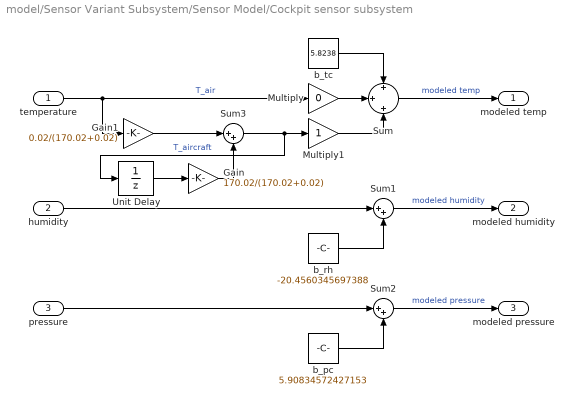
== system model/Sensor Variant Subsystem/Sensor Model/Cockpit sensor subsystem ==
  temperature : Inport
  humidity : Inport  Port=2
  pressure : Inport  Port=3
  Gain : Gain  Gain=170.02/(170.02+0.02)
  Gain1 : Gain  Gain=0.02/(170.02+0.02)
  Multiply : Gain  Gain=0
  Multiply1 : Gain
  Sum : Sum  Inputs=+|+|+
  Sum1 : Sum  Inputs=|++
  Sum2 : Sum  Inputs=|++
  Sum3 : Sum  Inputs=|++
  Unit Delay : UnitDelay  InitialCondition=295.423  SampleTime=-1  HasFrameUpgradeWarning=on
  b_pc : Constant  Value=5.90834572427153
  b_rh : Constant  Value=-20.4560345697388
  b_tc : Constant  Value=5.8238
  modeled temp : Outport
  modeled humidity : Outport  Port=2
  modeled pressure : Outport  Port=3
  wires:
  Multiply1/1 -> Sum/3
  Multiply/1 -> Sum/2
  temperature/1 -> Multiply/1, Gain1/1  "T_air"
  Sum/1 -> modeled temp/1  "modeled temp"
  pressure/1 -> Sum2/1
  b_pc/1 -> Sum2/2
  Sum2/1 -> modeled pressure/1  "modeled pressure"
  Sum1/1 -> modeled humidity/1  "modeled humidity"
  b_rh/1 -> Sum1/2
  humidity/1 -> Sum1/1
  Gain1/1 -> Sum3/1
  Sum3/1 -> Multiply1/1, Unit Delay/1  "T_aircraft"
  Unit Delay/1 -> Gain/1
  Gain/1 -> Sum3/2
  b_tc/1 -> Sum/1

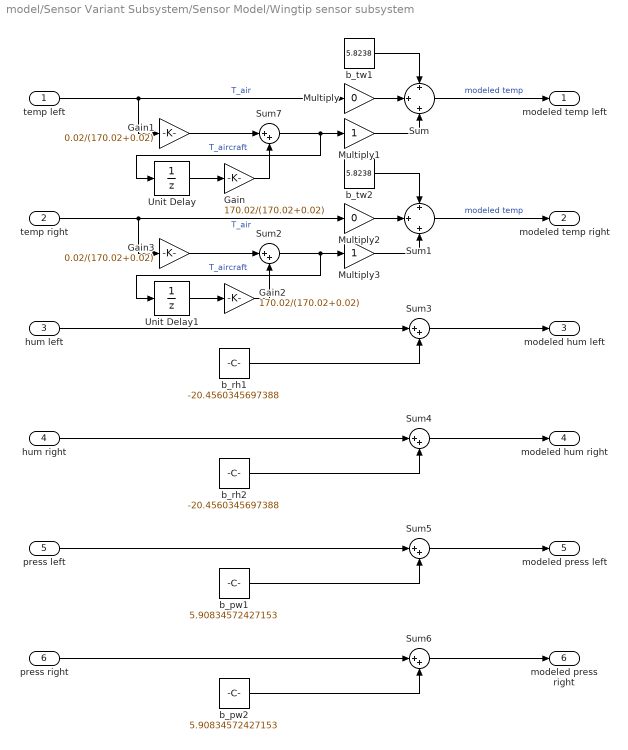
== system model/Sensor Variant Subsystem/Sensor Model/Wingtip sensor subsystem ==
  temp left : Inport
  temp right : Inport  Port=2
  hum left : Inport  Port=3
  hum right : Inport  Port=4
  press left : Inport  Port=5
  press right : Inport  Port=6
  Gain : Gain  Gain=170.02/(170.02+0.02)
  Gain1 : Gain  Gain=0.02/(170.02+0.02)
  Gain2 : Gain  Gain=170.02/(170.02+0.02)
  Gain3 : Gain  Gain=0.02/(170.02+0.02)
  Multiply : Gain  Gain=0
  Multiply1 : Gain
  Multiply2 : Gain  Gain=0
  Multiply3 : Gain
  Sum : Sum  Inputs=+|+|+
  Sum1 : Sum  Inputs=+|+|+
  Sum{2..7} (6 alike) : Sum  Inputs=|++
  Unit Delay : UnitDelay  InitialCondition=292  SampleTime=-1  HasFrameUpgradeWarning=on
  Unit Delay1 : UnitDelay  InitialCondition=292  SampleTime=-1  HasFrameUpgradeWarning=on
  b_pw1 : Constant  Value=5.90834572427153
  b_pw2 : Constant  Value=5.90834572427153
  b_rh1 : Constant  Value=-20.4560345697388
  b_rh2 : Constant  Value=-20.4560345697388
  b_tw1 : Constant  Value=5.8238
  b_tw2 : Constant  Value=5.8238
  modeled temp left : Outport
  modeled temp right : Outport  Port=2
  modeled hum left : Outport  Port=3
  modeled hum right : Outport  Port=4
  modeled press left : Outport  Port=5
  modeled press right : Outport  Port=6
  wires:
  Sum3/1 -> modeled hum left/1
  b_rh1/1 -> Sum3/2
  hum left/1 -> Sum3/1
  Sum4/1 -> modeled hum right/1
  b_rh2/1 -> Sum4/2
  hum right/1 -> Sum4/1
  b_pw1/1 -> Sum5/2
  press left/1 -> Sum5/1
  Sum5/1 -> modeled press left/1
  b_pw2/1 -> Sum6/2
  press right/1 -> Sum6/1
  Sum6/1 -> modeled press right/1
  b_tw1/1 -> Sum/1
  temp left/1 -> Multiply/1, Gain1/1  "T_air"
  Unit Delay/1 -> Gain/1
  Sum/1 -> modeled temp left/1  "modeled temp"
  Gain1/1 -> Sum7/1
  Multiply/1 -> Sum/2
  Gain/1 -> Sum7/2
  Multiply1/1 -> Sum/3
  Sum7/1 -> Multiply1/1, Unit Delay/1  "T_aircraft"
  b_tw2/1 -> Sum1/1
  temp right/1 -> Multiply2/1, Gain3/1  "T_air"
  Unit Delay1/1 -> Gain2/1
  Sum1/1 -> modeled temp right/1  "modeled temp"
  Gain3/1 -> Sum2/1
  Multiply2/1 -> Sum1/2
  Gain2/1 -> Sum2/2
  Multiply3/1 -> Sum1/3
  Sum2/1 -> Multiply3/1, Unit Delay1/1  "T_aircraft"

== matlab function model/Thermal Locator/NED Gradient direction ==
  data: grad input; dir output; euler_angles input
function dir = fcn(grad,euler_angles)

    z = grad(1) + grad(1)*1i;
    theta = angle(z) + euler_angles(3); % NED direction of gradient
    rho = 1000*abs(z); % scaled norm of gradient
 dir = [theta rho];

== matlab function model/Thermal Model ==
  data: T output size=[1 3] [1..1]; RH output size=[1 3]; p output size=[1 3]; lat input size=1; lon input size=1; alt input; euler_angles input; sounding_buses parameter Bus: sounding; updrafts parameter
function [T,RH,p] = updraft_model(lat,lon,alt, euler_angles, sounding_buses,updrafts)
    
% This block serves as a wrapper for the thermal_updraft.m function.
% Inputs: Aircraft position, euler angles, array of sounding buses, 
%         array of updraft locations
% Outputs: Temperature, relative humidity, pressure at the
%           [center, left wingtip, right wingtip] of the aircraft

   
    %% Call thermal model function
    if size(updrafts,1) % if there are updrafts

        % Call thermal model function
        [T,~,p,RH] = thermal_model(lat,lon,alt,euler_angles,updrafts,sounding_buses);
        T = T(1:3);
        p = p(1:3);
        RH = RH(1:3);
    else
        % Supress simulink coder error
        T = [0 0 0];
        p = [0 0 0];
        RH = [0 0 0];
    end

end

== matlab function model/Thermal Locator/calculate vpt ==
  data: T input; vpt output; RH input; p input
function vpt = virtual_potential_temperature(T, RH, p)
% virtual_potential_temperature Calculate the virtual potential temperature.
%
%   vpt = virtual_potential_temperature(T, RH, P) computes the virtual 
%   potential temperature given the temperature (T) in kelvin, relative 
%   humidity (RH) in percentage, and pressure (P) in pascals.
%
%   The function uses the August-Roche-Magnus equation to calculate the 
%   saturated vapor pressure.
%
%   Inputs:
%       T  - temperature in kelvin
%       RH - relative humidity in percentage
%       P  - pressure in pascals
%
%   Outputs:
%       vpt - virtual potential temperature in kelvin

    theta = T*(100000/p)^0.286; % potential temperature
    esat = 6.1094 * exp(17.625 * (T - 273.15)/(T - 273.15 + 243.04)); % saturated vapor pressure hPa
    e = RH * esat / 100; % vapor pressure hPa
    r = 0.622 * e/(p-e); % mixing ratio, unitless
    
    vpt = theta*(1+0.61*r); % virtual potential temperature in K
end

== matlab function model/Thermal Locator/calculate vpt1 ==
  data: T input; vpt output; RH input; p input
function vpt = virtual_potential_temperature(T, RH, p)
% virtual_potential_temperature Calculate the virtual potential temperature.
%
%   vpt = virtual_potential_temperature(T, RH, P) computes the virtual 
%   potential temperature given the temperature (T) in kelvin, relative 
%   humidity (RH) in percentage, and pressure (P) in pascals.
%
%   The function uses the August-Roche-Magnus equation to calculate the 
%   saturated vapor pressure.
%
%   Inputs:
%       T  - temperature in kelvin
%       RH - relative humidity in percentage
%       P  - pressure in pascals
%
%   Outputs:
%       vpt - virtual potential temperature in kelvin

    theta = T*(100000/p)^0.286; % potential temperature
    esat = 6.1094 * exp(17.625 * (T - 273.15)/(T - 273.15 + 243.04)); % saturated vapor pressure hPa
    e = RH * esat / 100; % vapor pressure hPa
    r = 0.622 * e/(p-e); % mixing ratio, unitless
    
    vpt = theta*(1+0.61*r); % virtual potential temperature in K
end

== matlab function model/Thermal Locator/calculate vpt2 ==
  data: T input; vpt output; RH input; p input
function vpt = virtual_potential_temperature(T, RH, p)
% virtual_potential_temperature Calculate the virtual potential temperature.
%
%   vpt = virtual_potential_temperature(T, RH, P) computes the virtual 
%   potential temperature given the temperature (T) in kelvin, relative 
%   humidity (RH) in percentage, and pressure (P) in pascals.
%
%   The function uses the August-Roche-Magnus equation to calculate the 
%   saturated vapor pressure.
%
%   Inputs:
%       T  - temperature in kelvin
%       RH - relative humidity in percentage
%       P  - pressure in pascals
%
%   Outputs:
%       vpt - virtual potential temperature in kelvin

    theta = T*(100000/p)^0.286; % potential temperature
    esat = 6.1094 * exp(17.625 * (T - 273.15)/(T - 273.15 + 243.04)); % saturated vapor pressure hPa
    e = RH * esat / 100; % vapor pressure hPa
    r = 0.622 * e/(p-e); % mixing ratio, unitless
    
    vpt = theta*(1+0.61*r); % virtual potential temperature in K
end

== matlab function model/Thermal Locator/body-fixed frame gradient ==
  data: vpt input; F output
function F = gradient(vpt)

F = thermal_gradient(vpt);

end
